simulink model "flyback_nonideal"  (R2022b)
settings: Solver=VariableStepAuto  StartTime=0.0  StopTime=0.2  RelTol=1e-3
libraries: spsSeriesRLCBranchLib x9, spsCurrentMeasurementLib x4, spsMeanLib x4, spsDiodeLib x2, spsVoltageMeasurementLib x2, spsDCVoltageSourceLib x1, spsLinearTransformerLib x1, spsMosfetLib x1, simulink x1, spsVariableRatioTransformerLib x1, sps_lib x1
settings Model: Creator=Mehmet Emre Doğan  LastModifiedBy=meteh

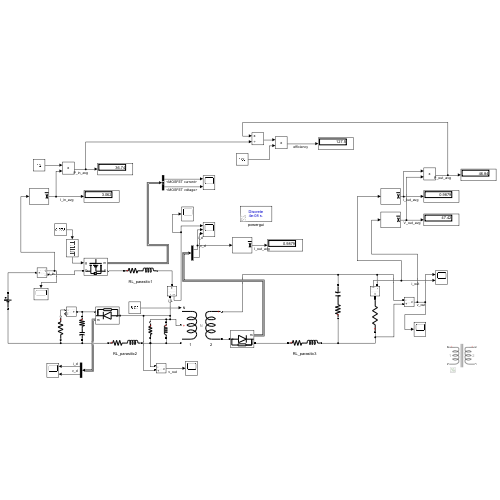
[thumbnail: Simulink's stored preview of the top-level diagram]
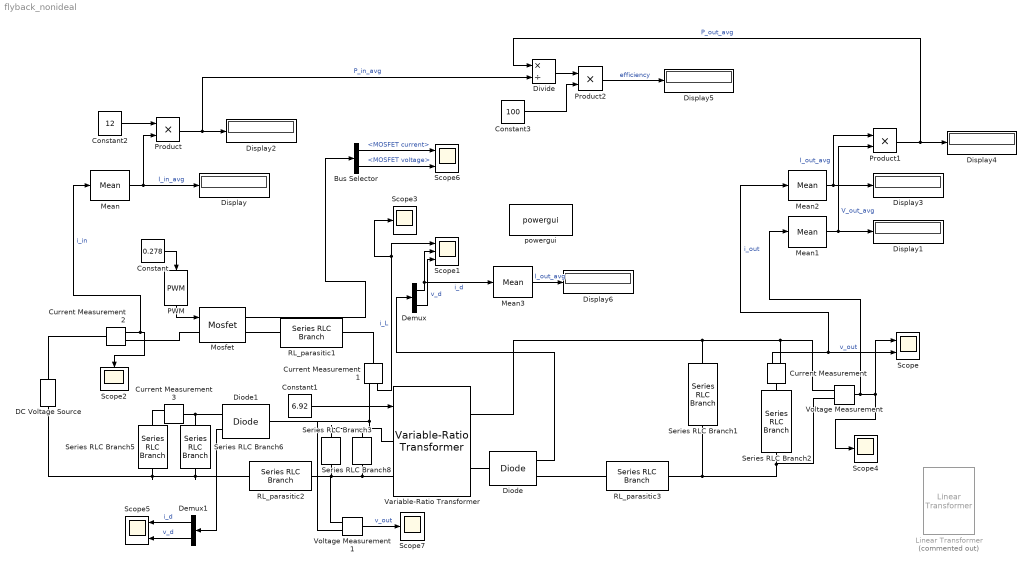
== system flyback_nonideal ==
  Bus Selector : BusSelector  OutputSignals=MOSFET current,MOSFET voltage
  Constant : Constant  Value=0.278
  Constant1 : Constant  Value=6.92
  Constant2 : Constant  Value=12
  Constant3 : Constant  Value=100
  Current Measurement{,1..3} (4 alike) : spsCurrentMeasurementLib/Current Measurement  PhasorSimulation=off  OutputType=Complex  PSBequivalent=0
  DC Voltage Source : spsDCVoltageSourceLib/DC Voltage Source  Amplitude=18  Measurements=None
  Demux : Demux  Outputs=2
  Demux1 : Demux  Outputs=2
  Diode : spsDiodeLib/Diode  Ron=0.001  Lon=0  Vf=0.5e-3  IC=0  UseSnubber=0  Rs=500e3  Cs=250e-9  Measurements=on
  Diode1 : spsDiodeLib/Diode  Ron=0.001  Lon=0  Vf=0.4e-3  IC=0  UseSnubber=0  Rs=500e3  Cs=250e-9  Measurements=on
  Display{,1..6} (7 alike) : Display
  Divide : Product  Inputs=*/
  Linear Transformer : spsLinearTransformerLib/Linear Transformer  Commented=on  UNITS=SI  NominalPower=[100 100e3]  winding1=[12 10.48e-3 56e-9]  winding2=[48 252.6e-3 56e-9]  ThreeWindings=off  winding3=[3.15e+05 0.7938 0.084225]  RmLm=[6.75, 8e-6]  Measurements=None  DataType=on
  Mean{,1..3} (4 alike) : spsMeanLib/Mean  Freq=100e3  Vinit=0  Ts=0
  Mosfet : spsMosfetLib/Mosfet  Ron=3.6e-3  Lon=0  Rd=0.01e-3  Vfd=0  IC=0  Rs=1e5  Cs=inf  Measurements=on
  PWM : simulink/Discontinuities/PWM  DisableCoverage=on  Period=1/(100e3)  InitialDelay=0  DisallowZeroDutyCycle=on  RunAtFixedTimeIntervals=off  SampleTime=0.1
  Product : Product
  Product1 : Product
  Product2 : Product
  RL_parasitic1 : spsSeriesRLCBranchLib/Series RLC Branch  LConnTagsString=__new0  RConnTagsString=__new0  BranchType=RL  Resistance=5e-3  Inductance=10e-9  SetiL0=off  InitialCurrent=0  Capacitance=10e-9  Setx0=off  InitialVoltage=0  Measurements=None
  RL_parasitic2 : spsSeriesRLCBranchLib/Series RLC Branch  LConnTagsString=__new0  RConnTagsString=__new0  BranchType=RL  Resistance=5e-3  Inductance=10e-9  SetiL0=off  InitialCurrent=0  Capacitance=10e-9  Setx0=off  InitialVoltage=0  Measurements=None
  RL_parasitic3 : spsSeriesRLCBranchLib/Series RLC Branch  LConnTagsString=__new0  RConnTagsString=__new0  BranchType=RL  Resistance=252e-3  Inductance=252e-9  SetiL0=off  InitialCurrent=0  Capacitance=1e-6  Setx0=off  InitialVoltage=0  Measurements=None
  Scope : Scope  NumInputPorts=2
  Scope1 : Scope  NumInputPorts=3
  Scope{2..4,7} (4 alike) : Scope
  Scope5 : Scope  NumInputPorts=2
  Scope6 : Scope  NumInputPorts=2
  Series RLC Branch1 : spsSeriesRLCBranchLib/Series RLC Branch  LConnTagsString=__new0  RConnTagsString=__new0  BranchType=RC  Resistance=10e-3  Inductance=1e-3  SetiL0=off  InitialCurrent=0  Capacitance=100e-6  Setx0=off  InitialVoltage=0  Measurements=None
  Series RLC Branch2 : spsSeriesRLCBranchLib/Series RLC Branch  LConnTagsString=__new0  RConnTagsString=__new0  BranchType=R  Resistance=48  Inductance=1e-3  SetiL0=off  InitialCurrent=0  Capacitance=1e-6  Setx0=off  InitialVoltage=0  Measurements=None
  Series RLC Branch3 : spsSeriesRLCBranchLib/Series RLC Branch  LConnTagsString=__new0  RConnTagsString=__new0  BranchType=L  Resistance=1  Inductance=8e-6  SetiL0=off  InitialCurrent=0  Capacitance=52e-6  Setx0=off  InitialVoltage=0  Measurements=None
  Series RLC Branch5 : spsSeriesRLCBranchLib/Series RLC Branch  LConnTagsString=__new0  RConnTagsString=__new0  BranchType=R  Resistance=60  Inductance=10e-9  SetiL0=off  InitialCurrent=0  Capacitance=10e-9  Setx0=off  InitialVoltage=0  Measurements=None
  Series RLC Branch6 : spsSeriesRLCBranchLib/Series RLC Branch  LConnTagsString=__new0  RConnTagsString=__new0  BranchType=RC  Resistance=1e-3  Inductance=10e-9  SetiL0=off  InitialCurrent=0  Capacitance=2.2e-6  Setx0=off  InitialVoltage=0  Measurements=None
  Series RLC Branch8 : spsSeriesRLCBranchLib/Series RLC Branch  LConnTagsString=__new0  RConnTagsString=__new0  BranchType=R  Resistance=65.1  Inductance=8e-6  SetiL0=off  InitialCurrent=0  Capacitance=52e-6  Setx0=off  InitialVoltage=0  Measurements=None
  Variable-Ratio Transformer : spsVariableRatioTransformerLib/Variable-Ratio Transformer
      settings: LibrarySourceBlock=|
      | sps_lib/Passives/Variable-Ratio
      | Transformer
  Voltage Measurement : spsVoltageMeasurementLib/Voltage Measurement  PhasorSimulation=off  OutputType=Complex  PSBequivalent=0
  Voltage Measurement1 : spsVoltageMeasurementLib/Voltage Measurement  PhasorSimulation=off  OutputType=Complex  PSBequivalent=0
  powergui : sps_lib/powergui  Priority=1  SimulationMode=Discrete  SampleTime=40e-9  frequency=60  Iterations=50  frequencyindice=0  Pbase=100e6  ErrMax=1e-4  UnitsV=kV  UnitsW=MW  buscounter=0  FunctionMessages=off  echomessages=off  EnableUseOfTLC=off  CurrentSourceSwitches=on  DisableSnubberDevices=off  DisableRonSwitches=off  DisableVfSwitches=off  DisplayEquations=off  AutomaticDiscreteSolvers=off  SolverType=Tustin/Backward Euler (TBE)  Interpol=off  ExternalGateDelay=off  methode=off  Ts=100  x0status=blocks  SPID=on  SwTol=0  HookPort=off  NonlinearTolerance=1e-4  nMaxIteration=100  ContinueOnMaxIteration=off  RestoreLinks=warning  ResistiveCurrentMeasurement=off  Frange=[0:2:500]  Ylog=off  Xlog=on  ShowGrid=off  save=off  variable=ZData  structure=0  ZoomFFT=off  StartTime=0.0  cycles=1  DisplayStyle=1  fundamental=60  FreqAxis=off  MaxFrequency=1000  frequencyindicesteady=1  RmsSteady=1  display=off
  wires:
  Constant/1 -> PWM/1
  PWM/1 -> Mosfet/1
  Voltage Measurement/1 -> Mean1/1, Scope/1, Scope4/1  "v_out"
  Current Measurement/1 -> Scope/2, Mean2/1  "i_out"
  Current Measurement1/1 -> Scope3/1, Scope1/1  "i_L"
  Current Measurement2/1 -> Mean/1, Scope2/1  "i_in"
  Demux/1 -> Mean3/1, Scope1/2  "i_d"
  Demux/2 -> Scope1/3  "v_d"
  Diode/1 -> Demux/1
  Constant1/1 -> Variable-Ratio Transformer/1
  Diode1/1 -> Demux1/1
  Demux1/1 -> Scope5/1  "i_d"
  Demux1/2 -> Scope5/2  "v_d"
  Mosfet/1 -> Bus Selector/1
  Bus Selector/1 -> Scope6/1  "<MOSFET current>"
  Bus Selector/2 -> Scope6/2  "<MOSFET voltage>"
  Mean/1 -> Product/2, Display/1  "I_in_avg"
  Mean1/1 -> Product1/2, Display1/1  "V_out_avg"
  Constant2/1 -> Product/1
  Product/1 -> Divide/2, Display2/1  "P_in_avg"
  Mean2/1 -> Product1/1, Display3/1  "I_out_avg"
  Product1/1 -> Divide/1, Display4/1  "P_out_avg"
  Voltage Measurement1/1 -> Scope7/1  "v_out"
  Product2/1 -> Display5/1  "efficiency"
  Constant3/1 -> Product2/2
  Divide/1 -> Product2/1
  Mean3/1 -> Display6/1  "I_out_avg"
  connections:
  Mosfet/LConn1 -- Current Measurement2/RConn1
  Series RLC Branch2/LConn1 -- RL_parasitic3/RConn1 -- Series RLC Branch1/LConn1 -- Voltage Measurement/LConn1
  Current Measurement1/RConn1 -- Voltage Measurement1/LConn1 -- Diode1/LConn1 -- Series RLC Branch8/LConn1 -- Series RLC Branch3/LConn1 -- Variable-Ratio Transformer/LConn1
  Series RLC Branch2/RConn1 -- Current Measurement/LConn1
  Series RLC Branch8/RConn1 -- Voltage Measurement1/LConn2 -- RL_parasitic2/RConn1 -- Variable-Ratio Transformer/LConn2 -- Series RLC Branch3/RConn1
  Voltage Measurement/LConn2 -- Current Measurement/RConn1 -- Variable-Ratio Transformer/RConn1 -- Series RLC Branch1/RConn1
  Variable-Ratio Transformer/RConn2 -- Diode/LConn1
  RL_parasitic3/LConn1 -- Diode/RConn1
  Series RLC Branch6/LConn1 -- Diode1/RConn1 -- Current Measurement3/LConn1
  DC Voltage Source/RConn1 -- Current Measurement2/LConn1
  Series RLC Branch6/RConn1 -- DC Voltage Source/LConn1 -- Series RLC Branch5/RConn1 -- RL_parasitic2/LConn1
  RL_parasitic1/LConn1 -- Mosfet/RConn1
  RL_parasitic1/RConn1 -- Current Measurement1/LConn1
  Current Measurement3/RConn1 -- Series RLC Branch5/LConn1
